simulink model "PCM"  (R2018a)
settings: Solver=VariableStepAuto  StartTime=0.0  StopTime=10.0  RelTol=1e-3
libraries: commutil2 x1, dspquant2 x1
settings Model: Creator=shahb  LastModifiedBy=shahb

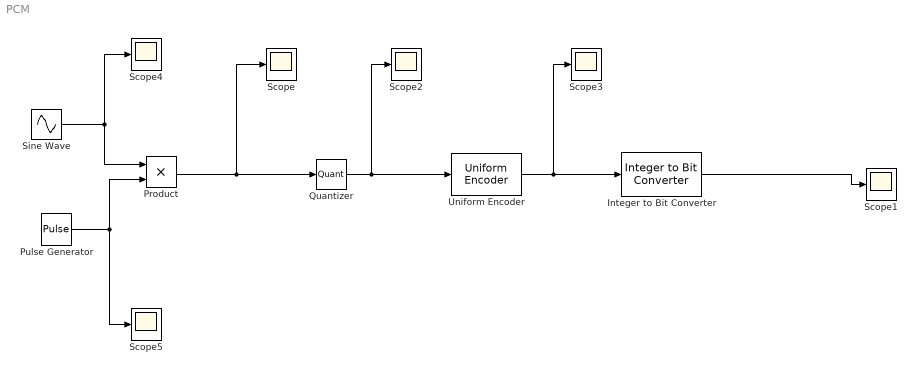
== system PCM ==
  Integer to Bit Converter : commutil2/Integer to Bit Converter  nbits=32  signedInputValues=Unsigned  bitOrder=MSB first  outDtype=Inherit via internal rule
  Product : Product
  Pulse Generator : DiscretePulseGenerator  PulseType=Time based  Period=0.1  PulseWidth=5
  Quantizer : Quantizer
  Scope{,1..5} (6 alike) : Scope
  Sine Wave : Sin  SampleTime=0
  Uniform Encoder : dspquant2/Uniform Encoder  peak=1  bits=8  otype=Unsigned integer
      settings: SourceProductName=DSP System Toolbox
  wires:
  Product/1 -> Quantizer/1, Scope/1
  Quantizer/1 -> Scope2/1, Uniform Encoder/1
  Uniform Encoder/1 -> Scope3/1, Integer to Bit Converter/1
  Integer to Bit Converter/1 -> Scope1/1
  Sine Wave/1 -> Scope4/1, Product/1
  Pulse Generator/1 -> Scope5/1, Product/2
